simulink model "DcMotor_Control"  (R2018a)
settings: Solver=VariableStepAuto  StartTime=t(1)  StopTime=t(end)  RelTol=1e-3
undefined symbols (not defined in the file): B, id_num_L, Ts
libraries: simulink x1
settings Model: Creator=peppe  LastModifiedBy=peppe

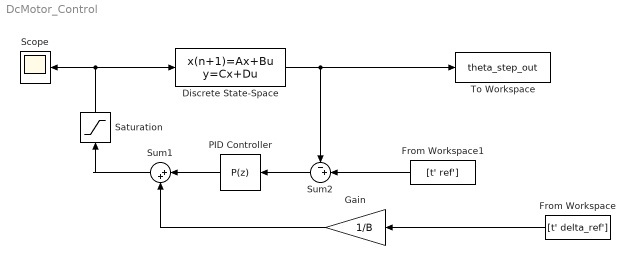
== system DcMotor_Control ==
  Discrete State-Space : DiscreteStateSpace  B=id_num_L(2)  D=0  SampleTime=Ts
  From Workspace : FromWorkspace  VariableName=[t' delta_ref']  SampleTime=Ts
  From Workspace1 : FromWorkspace  VariableName=[t' ref']  SampleTime=Ts
  Gain : Gain  Gain=1/B
  PID Controller : simulink/Continuous/PID Controller  Controller=P  TimeDomain=Discrete-time  SampleTime=Ts  IntegratorMethod=Forward Euler  FilterMethod=Forward Euler  Form=Parallel  UseFilter=off  ControllerParametersSource=internal  P=4.30269668915073  I=0  D=0  N=100  InitialConditionSource=internal  InitialConditionForIntegrator=0  InitialConditionForFilter=0  ExternalReset=none  LimitOutput=off  UpperSaturationLimit=inf  LowerSaturationLimit=-inf  LinearizeAsGain=on  AntiWindupMode=none  Kb=1  TrackingMode=off  Kt=1  PParamMin=[]  PParamMax=[]  IParamMin=[]  IParamMax=[]  DParamMin=[]  DParamMax=[]  NParamMin=[]  NParamMax=[]  KbParamMin=[]  KbParamMax=[]  KtParamMin=[]  KtParamMax=[]  POutMin=[]  POutMax=[]  IOutMin=[]  IOutMax=[]  DOutMin=[]  DOutMax=[]  NOutMin=[]  NOutMax=[]  KbOutMin=[]  KbOutMax=[]  KtOutMin=[]  KtOutMax=[]  IntegratorOutMin=[]  IntegratorOutMax=[]  FilterOutMin=[]  FilterOutMax=[]  SumOutMin=[]  SumOutMax=[]  SumI1OutMin=[]  SumI1OutMax=[]  SumI2OutMin=[]  SumI2OutMax=[]  SumI3OutMin=[]  SumI3OutMax=[]  SumDOutMin=[]  SumDOutMax=[]  SaturationOutMin=[]  SaturationOutMax=[]  IntegratorContinuousStateAttributes=''  IntegratorStateMustResolveToSignalObject=off  IntegratorRTWStateStorageClass=Auto  FilterContinuousStateAttributes=''  FilterStateMustResolveToSignalObject=off  FilterRTWStateStorageClass=Auto  DifferentiatorICPrevScaledInput=0  DifferentiatorOutMin=[]  DifferentiatorOutMax=[]  FilterDiffOutCoefMin=[]  FilterDiffOutCoefMax=[]  SumDenOutMin=[]  SumDenOutMax=[]  SumNumOutMin=[]  SumNumOutMax=[]  ReciprocalOutMin=[]  ReciprocalOutMax=[]  DivideOutMin=[]  DivideOutMax=[]  TunerSelectOption=Transfer Function Based (PID Tuner App)
  Saturation : Saturate  UpperLimit=5.5  LowerLimit=-5.5
  Scope : Scope
  Sum1 : Sum  Inputs=|++
  Sum2 : Sum  Inputs=-+|
  To Workspace : ToWorkspace  VariableName=theta_step_out  SaveFormat=Timeseries  SampleTime=Ts
  wires:
  Discrete State-Space/1 -> Sum2/1, To Workspace/1
  From Workspace/1 -> Gain/1
  Gain/1 -> Sum1/2
  Sum2/1 -> PID Controller/1
  Sum1/1 -> Saturation/1
  Saturation/1 -> Scope/1, Discrete State-Space/1
  PID Controller/1 -> Sum1/1
  From Workspace1/1 -> Sum2/2
